simulink model "rocket_6dof_sim"  (R2024a)
settings: Solver=FixedStepAuto  StartTime=0.0  StopTime=35  RelTol=1e-8  AbsTol=1e-8
values from neighbouring files (symbols this model uses):
  p = c(1)+c(2)*tau+c(3)*tau.^2+c(4)*tau.^3+c(5)*tau.^4+c(6)*tau.^5    [envelope_mais_monte_carlo_final.m]    (also in init_mpc.m = falcon9_params(); init_sim.m = falcon9_params(); run_scurve.m = falcon9_params(); simulate_openloop.m = falcon9_params())
  x0_sim = [ic.x0; ic.y0; ic.h0; 0; 0; ic.vz0;                ic.phi0; ic.theta0; 0; 0; ic.q0; 0; ic.m0]    [envelope_mais_monte_carlo_final.m]    (also in init_mpc.m = [p.x0; p.y0; p.h0; init_sim.m = [p.x0)
libraries: simulink_extras x6, simulink x2
settings Model: SimulationMode=accelerator  Creator=marin  LastModifiedBy=marin
settings DataIOCC: SaveFormat=Array
settings OptimizationCC: BlockReduction=off  DefaultParameterBehavior=Inlined  BufferReuse=off

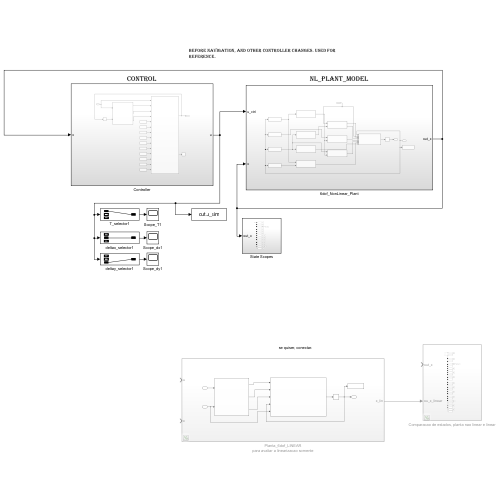
[thumbnail: Simulink's stored preview of the top-level diagram]
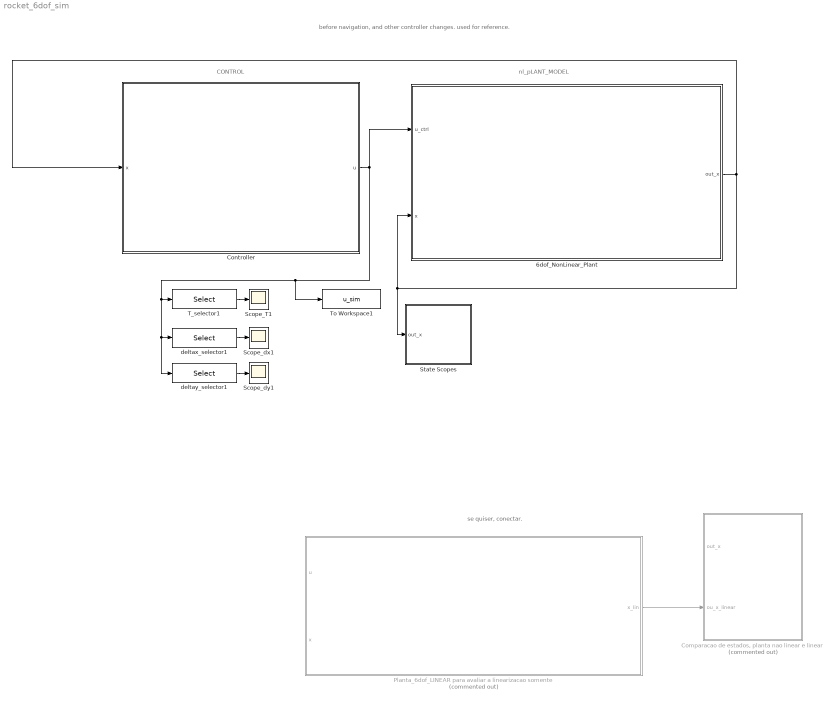
== system rocket_6dof_sim ==
  note: se quiser, conectar.
  note: CONTROL
  note: nl_pLANT_MODEL
  note: before navigation, and other controller changes. used for reference.
  6dof_NonLinear_Plant : Subsystem
  "Comparacao de estados, planta nao linear e linear" : Subsystem  Commented=on
  Controller : Subsystem
  Planta_6dof_LINEAR para avaliar a linearizacao somente : Subsystem  Commented=on
  Scope_T1 : Scope
  Scope_dx1 : Scope
  Scope_dy1 : Scope
  State Scopes : Subsystem
  T_selector1 : Selector  InputPortWidth=3  IndexOptions=Index vector (dialog)  Indices=1  OutputSizes=1
  To Workspace1 : ToWorkspace  VariableName=u_sim  SaveFormat=Timeseries  SampleTime=-1
  deltax_selector1 : Selector  InputPortWidth=3  IndexOptions=Index vector (dialog)  Indices=2  OutputSizes=1
  deltay_selector1 : Selector  InputPortWidth=3  IndexOptions=Index vector (dialog)  Indices=3  OutputSizes=1
  wires:
  deltax_selector1/1 -> Scope_dx1/1
  6dof_NonLinear_Plant/1(out_x) -> Controller/1(x), 6dof_NonLinear_Plant/2(x), State Scopes/1(out_x)
  Controller/1(u) -> 6dof_NonLinear_Plant/1(u_ctrl), deltay_selector1/1, deltax_selector1/1, T_selector1/1, To Workspace1/1
  deltay_selector1/1 -> Scope_dy1/1
  T_selector1/1 -> Scope_T1/1
  Planta_6dof_LINEAR para avaliar a linearizacao somente/1(x_lin) -> "Comparacao de estados, planta nao linear e linear"/2(ou_x_linear)

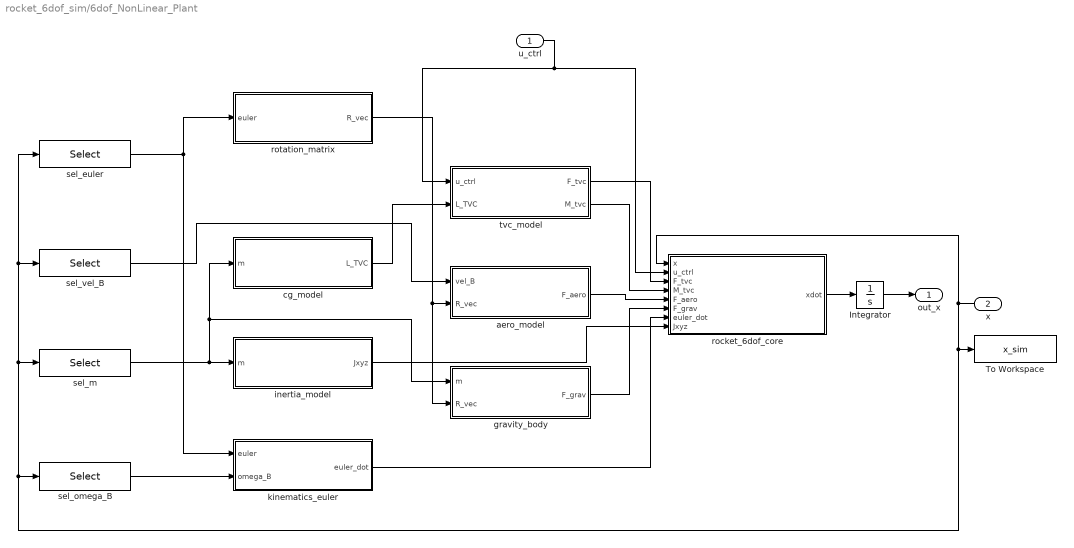
== system rocket_6dof_sim/6dof_NonLinear_Plant ==
  u_ctrl : Inport
  x : Inport  Port=2
  Integrator : Integrator  InitialCondition=x0_sim
  To Workspace : ToWorkspace  VariableName=x_sim  SaveFormat=Timeseries  SampleTime=0.01
  aero_model : MATLAB Function  TreatAsAtomicUnit=on
  cg_model : MATLAB Function  TreatAsAtomicUnit=on
  gravity_body : MATLAB Function  TreatAsAtomicUnit=on
  inertia_model : MATLAB Function  TreatAsAtomicUnit=on
  kinematics_euler : MATLAB Function  TreatAsAtomicUnit=on
  rocket_6dof_core : MATLAB Function  TreatAsAtomicUnit=on
  rotation_matrix : MATLAB Function  TreatAsAtomicUnit=on
  sel_euler : Selector  InputPortWidth=13  IndexOptions=Index vector (dialog)  Indices=7:9  OutputSizes=1
  sel_m : Selector  InputPortWidth=13  IndexOptions=Index vector (dialog)  Indices=13  OutputSizes=1
  sel_omega_B : Selector  InputPortWidth=13  IndexOptions=Index vector (dialog)  Indices=10:12  OutputSizes=1
  sel_vel_B : Selector  InputPortWidth=13  IndexOptions=Index vector (dialog)  Indices=4:6  OutputSizes=1
  tvc_model : MATLAB Function  TreatAsAtomicUnit=on
  out_x : Outport
  wires:
  sel_vel_B/1 -> aero_model/1(vel_B)
  cg_model/1(L_TVC) -> tvc_model/2(L_TVC)
  inertia_model/1(Jxyz) -> rocket_6dof_core/8(Jxyz)
  x/1 -> To Workspace/1, sel_m/1, sel_vel_B/1, sel_euler/1, sel_omega_B/1, rocket_6dof_core/1(x)
  sel_m/1 -> cg_model/1(m), gravity_body/1(m), inertia_model/1(m)
  kinematics_euler/1(euler_dot) -> rocket_6dof_core/7(euler_dot)
  gravity_body/1(F_grav) -> rocket_6dof_core/6(F_grav)
  tvc_model/2(M_tvc) -> rocket_6dof_core/4(M_tvc)
  rotation_matrix/1(R_vec) -> gravity_body/2(R_vec), aero_model/2(R_vec)
  aero_model/1(F_aero) -> rocket_6dof_core/5(F_aero)
  u_ctrl/1 -> rocket_6dof_core/2(u_ctrl), tvc_model/1(u_ctrl)
  tvc_model/1(F_tvc) -> rocket_6dof_core/3(F_tvc)
  Integrator/1 -> out_x/1
  rocket_6dof_core/1(xdot) -> Integrator/1
  sel_omega_B/1 -> kinematics_euler/2(omega_B)
  sel_euler/1 -> rotation_matrix/1(euler), kinematics_euler/1(euler)

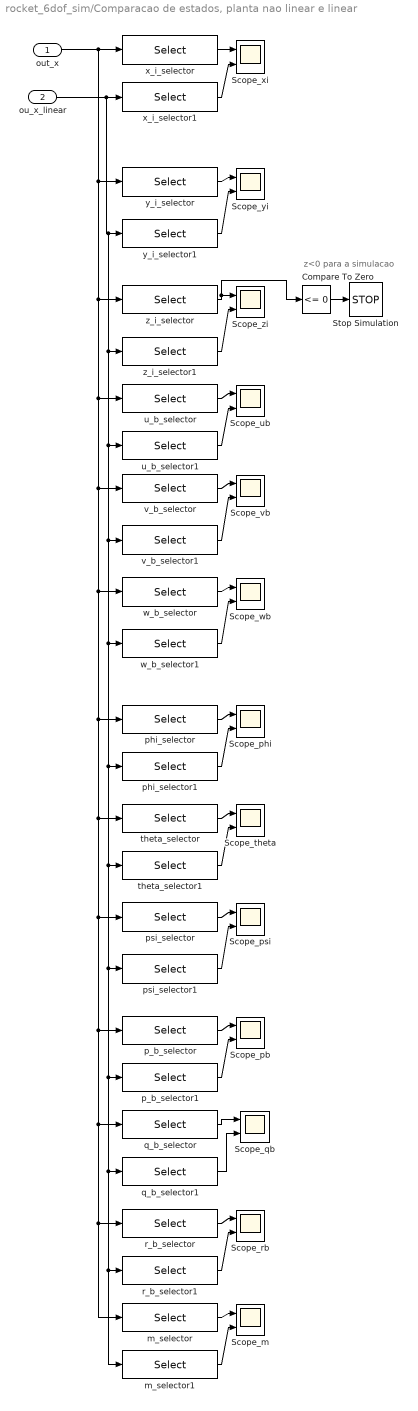
== system rocket_6dof_sim/Comparacao de estados, planta nao linear e linear ==
  note: z<0 para a simulacao
  out_x : Inport
  ou_x_linear : Inport  Port=2
  Compare To Zero : simulink/Logic and Bit Operations/Compare To Zero  relop=<=  OutDataTypeStr=boolean
  Scope_m : Scope  NumInputPorts=2
  Scope_pb : Scope  NumInputPorts=2
  Scope_phi : Scope  NumInputPorts=2
  Scope_psi : Scope  NumInputPorts=2
  Scope_qb : Scope  NumInputPorts=2
  Scope_rb : Scope  NumInputPorts=2
  Scope_theta : Scope  NumInputPorts=2
  Scope_ub : Scope  NumInputPorts=2
  Scope_vb : Scope  NumInputPorts=2
  Scope_wb : Scope  NumInputPorts=2
  Scope_xi : Scope  NumInputPorts=2
  Scope_yi : Scope  NumInputPorts=2
  Scope_zi : Scope  NumInputPorts=2
  Stop Simulation : Stop
  m_selector : Selector  InputPortWidth=13  IndexOptions=Index vector (dialog)  Indices=13  OutputSizes=1
  m_selector1 : Selector  InputPortWidth=13  IndexOptions=Index vector (dialog)  Indices=13  OutputSizes=1
  p_b_selector : Selector  InputPortWidth=13  IndexOptions=Index vector (dialog)  Indices=10  OutputSizes=1
  p_b_selector1 : Selector  InputPortWidth=13  IndexOptions=Index vector (dialog)  Indices=10  OutputSizes=1
  phi_selector : Selector  InputPortWidth=13  IndexOptions=Index vector (dialog)  Indices=7  OutputSizes=1
  phi_selector1 : Selector  InputPortWidth=13  IndexOptions=Index vector (dialog)  Indices=7  OutputSizes=1
  psi_selector : Selector  InputPortWidth=13  IndexOptions=Index vector (dialog)  Indices=9  OutputSizes=1
  psi_selector1 : Selector  InputPortWidth=13  IndexOptions=Index vector (dialog)  Indices=9  OutputSizes=1
  q_b_selector : Selector  InputPortWidth=13  IndexOptions=Index vector (dialog)  Indices=11  OutputSizes=1
  q_b_selector1 : Selector  InputPortWidth=13  IndexOptions=Index vector (dialog)  Indices=11  OutputSizes=1
  r_b_selector : Selector  InputPortWidth=13  IndexOptions=Index vector (dialog)  Indices=12  OutputSizes=1
  r_b_selector1 : Selector  InputPortWidth=13  IndexOptions=Index vector (dialog)  Indices=12  OutputSizes=1
  theta_selector : Selector  InputPortWidth=13  IndexOptions=Index vector (dialog)  Indices=8  OutputSizes=1
  theta_selector1 : Selector  InputPortWidth=13  IndexOptions=Index vector (dialog)  Indices=8  OutputSizes=1
  u_b_selector : Selector  InputPortWidth=13  IndexOptions=Index vector (dialog)  Indices=4  OutputSizes=1
  u_b_selector1 : Selector  InputPortWidth=13  IndexOptions=Index vector (dialog)  Indices=4  OutputSizes=1
  v_b_selector : Selector  InputPortWidth=13  IndexOptions=Index vector (dialog)  Indices=5  OutputSizes=1
  v_b_selector1 : Selector  InputPortWidth=13  IndexOptions=Index vector (dialog)  Indices=5  OutputSizes=1
  w_b_selector : Selector  InputPortWidth=13  IndexOptions=Index vector (dialog)  Indices=6  OutputSizes=1
  w_b_selector1 : Selector  InputPortWidth=13  IndexOptions=Index vector (dialog)  Indices=6  OutputSizes=1
  x_i_selector : Selector  InputPortWidth=13  IndexOptions=Index vector (dialog)  Indices=1  OutputSizes=1
  x_i_selector1 : Selector  InputPortWidth=13  IndexOptions=Index vector (dialog)  Indices=1  OutputSizes=1
  y_i_selector : Selector  InputPortWidth=13  IndexOptions=Index vector (dialog)  Indices=2  OutputSizes=1
  y_i_selector1 : Selector  InputPortWidth=13  IndexOptions=Index vector (dialog)  Indices=2  OutputSizes=1
  z_i_selector : Selector  InputPortWidth=13  IndexOptions=Index vector (dialog)  Indices=3  OutputSizes=1
  z_i_selector1 : Selector  InputPortWidth=13  IndexOptions=Index vector (dialog)  Indices=3  OutputSizes=1
  wires:
  u_b_selector/1 -> Scope_ub/1
  psi_selector/1 -> Scope_psi/1
  y_i_selector/1 -> Scope_yi/1
  q_b_selector/1 -> Scope_qb/1
  p_b_selector/1 -> Scope_pb/1
  phi_selector/1 -> Scope_phi/1
  v_b_selector/1 -> Scope_vb/1
  r_b_selector/1 -> Scope_rb/1
  w_b_selector/1 -> Scope_wb/1
  m_selector/1 -> Scope_m/1
  theta_selector/1 -> Scope_theta/1
  z_i_selector/1 -> Compare To Zero/1, Scope_zi/1
  out_x/1 -> v_b_selector/1, psi_selector/1, p_b_selector/1, q_b_selector/1, r_b_selector/1, m_selector/1, theta_selector/1, phi_selector/1, w_b_selector/1, u_b_selector/1, z_i_selector/1, y_i_selector/1, x_i_selector/1
  Compare To Zero/1 -> Stop Simulation/1
  y_i_selector1/1 -> Scope_yi/2
  z_i_selector1/1 -> Scope_zi/2
  u_b_selector1/1 -> Scope_ub/2
  v_b_selector1/1 -> Scope_vb/2
  w_b_selector1/1 -> Scope_wb/2
  phi_selector1/1 -> Scope_phi/2
  theta_selector1/1 -> Scope_theta/2
  psi_selector1/1 -> Scope_psi/2
  p_b_selector1/1 -> Scope_pb/2
  q_b_selector1/1 -> Scope_qb/2
  r_b_selector1/1 -> Scope_rb/2
  m_selector1/1 -> Scope_m/2
  ou_x_linear/1 -> m_selector1/1, r_b_selector1/1, q_b_selector1/1, p_b_selector1/1, psi_selector1/1, theta_selector1/1, phi_selector1/1, w_b_selector1/1, v_b_selector1/1, u_b_selector1/1, z_i_selector1/1, y_i_selector1/1, x_i_selector1/1
  x_i_selector/1 -> Scope_xi/1
  x_i_selector1/1 -> Scope_xi/2

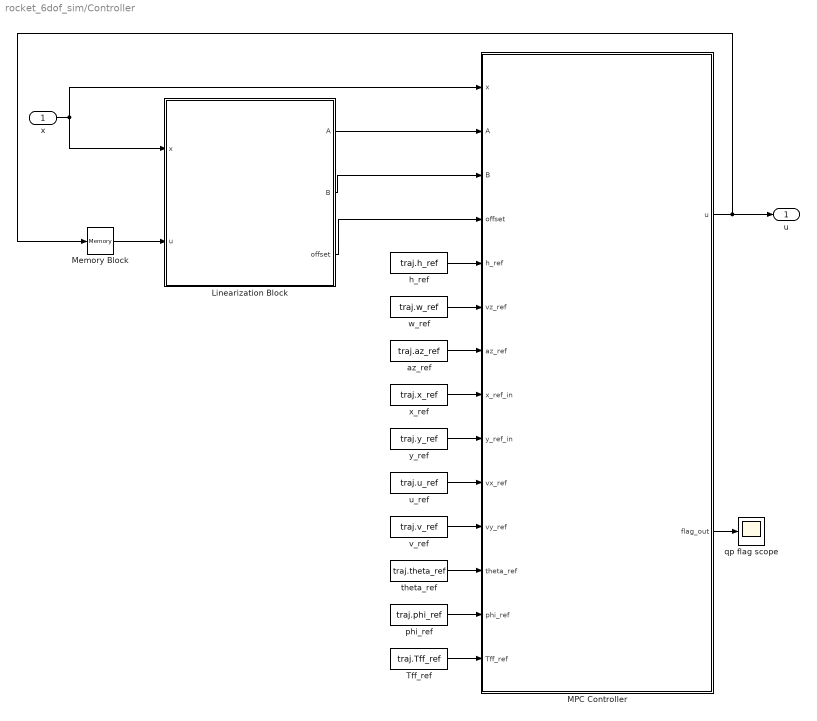
== system rocket_6dof_sim/Controller ==
  x : Inport
  Linearization Block : MATLAB Function  TreatAsAtomicUnit=on  SystemSampleTime=0.01
  MPC Controller : MATLAB Function  TreatAsAtomicUnit=on  SystemSampleTime=0.001
  Memory Block : Memory  InitialCondition=[p.T_min; 0; 0]
  Tff_ref : FromWorkspace  VariableName=traj.Tff_ref  OutputAfterFinalValue=Holding final value
  az_ref : FromWorkspace  VariableName=traj.az_ref  OutputAfterFinalValue=Holding final value
  h_ref : FromWorkspace  VariableName=traj.h_ref  OutputAfterFinalValue=Holding final value
  phi_ref : FromWorkspace  VariableName=traj.phi_ref  OutputAfterFinalValue=Holding final value
  qp flag scope : Scope
  theta_ref : FromWorkspace  VariableName=traj.theta_ref  OutputAfterFinalValue=Holding final value
  u_ref : FromWorkspace  VariableName=traj.u_ref
  v_ref : FromWorkspace  VariableName=traj.v_ref
  w_ref : FromWorkspace  VariableName=traj.w_ref
  x_ref : FromWorkspace  VariableName=traj.x_ref  OutputAfterFinalValue=Holding final value
  y_ref : FromWorkspace  VariableName=traj.y_ref  OutputAfterFinalValue=Holding final value
  u : Outport
  wires:
  y_ref/1 -> MPC Controller/9(y_ref_in)
  theta_ref/1 -> MPC Controller/12(theta_ref)
  Linearization Block/1(A) -> MPC Controller/2(A)
  h_ref/1 -> MPC Controller/5(h_ref)
  phi_ref/1 -> MPC Controller/13(phi_ref)
  MPC Controller/1(u) -> u/1, Memory Block/1
  x_ref/1 -> MPC Controller/8(x_ref_in)
  az_ref/1 -> MPC Controller/7(az_ref)
  Tff_ref/1 -> MPC Controller/14(Tff_ref)
  Linearization Block/2(B) -> MPC Controller/3(B)
  x/1 -> MPC Controller/1(x), Linearization Block/1(x)
  Linearization Block/3(offset) -> MPC Controller/4(offset)
  Memory Block/1 -> Linearization Block/2(u)
  MPC Controller/2(flag_out) -> qp flag scope/1
  u_ref/1 -> MPC Controller/10(vx_ref)
  w_ref/1 -> MPC Controller/6(vz_ref)
  v_ref/1 -> MPC Controller/11(vy_ref)

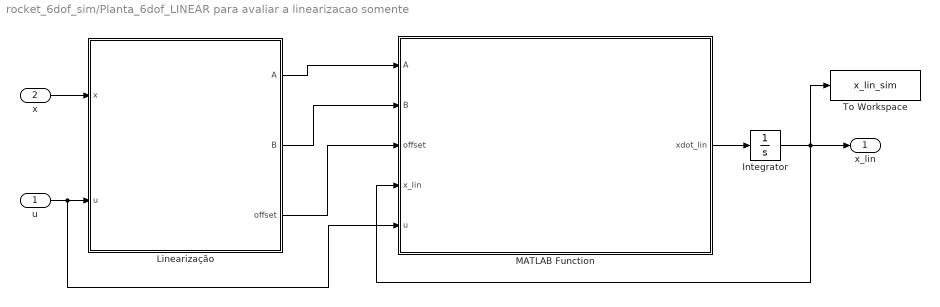
== system rocket_6dof_sim/Planta_6dof_LINEAR para avaliar a linearizacao somente ==
  u : Inport
  x : Inport  Port=2
  Integrator : Integrator  InitialCondition=x0_sim
  Linearização : MATLAB Function  TreatAsAtomicUnit=on  SystemSampleTime=0.3
  MATLAB Function : MATLAB Function  TreatAsAtomicUnit=on
  To Workspace : ToWorkspace  VariableName=x_lin_sim  SaveFormat=Timeseries  SampleTime=0.01
  x_lin : Outport
  wires:
  Linearização/1(A) -> MATLAB Function/1(A)
  Integrator/1 -> To Workspace/1, x_lin/1, MATLAB Function/4(x_lin)
  MATLAB Function/1(xdot_lin) -> Integrator/1
  Linearização/3(offset) -> MATLAB Function/3(offset)
  Linearização/2(B) -> MATLAB Function/2(B)
  u/1 -> MATLAB Function/5(u), Linearização/2(u)
  x/1 -> Linearização/1(x)

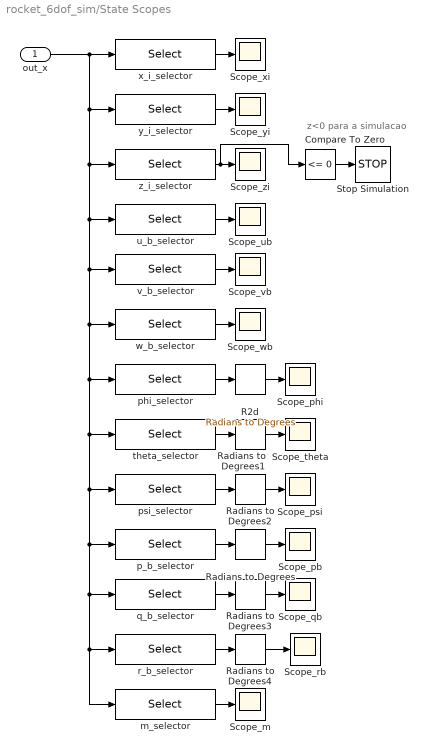
== system rocket_6dof_sim/State Scopes ==
  note: z<0 para a simulacao
  out_x : Inport
  Compare To Zero : simulink/Logic and Bit Operations/Compare To Zero  relop=<=  OutDataTypeStr=boolean
  R2d : simulink_extras/Transformations/Radians to Degrees
  Radians to Degrees{,1..4} (5 alike) : simulink_extras/Transformations/Radians to Degrees
  Scope_m : Scope
  Scope_pb : Scope
  Scope_phi : Scope
  Scope_psi : Scope
  Scope_qb : Scope
  Scope_rb : Scope
  Scope_theta : Scope
  Scope_ub : Scope
  Scope_vb : Scope
  Scope_wb : Scope
  Scope_xi : Scope
  Scope_yi : Scope
  Scope_zi : Scope
  Stop Simulation : Stop
  m_selector : Selector  InputPortWidth=13  IndexOptions=Index vector (dialog)  Indices=13  OutputSizes=1
  p_b_selector : Selector  InputPortWidth=13  IndexOptions=Index vector (dialog)  Indices=10  OutputSizes=1
  phi_selector : Selector  InputPortWidth=13  IndexOptions=Index vector (dialog)  Indices=7  OutputSizes=1
  psi_selector : Selector  InputPortWidth=13  IndexOptions=Index vector (dialog)  Indices=9  OutputSizes=1
  q_b_selector : Selector  InputPortWidth=13  IndexOptions=Index vector (dialog)  Indices=11  OutputSizes=1
  r_b_selector : Selector  InputPortWidth=13  IndexOptions=Index vector (dialog)  Indices=12  OutputSizes=1
  theta_selector : Selector  InputPortWidth=13  IndexOptions=Index vector (dialog)  Indices=8  OutputSizes=1
  u_b_selector : Selector  InputPortWidth=13  IndexOptions=Index vector (dialog)  Indices=4  OutputSizes=1
  v_b_selector : Selector  InputPortWidth=13  IndexOptions=Index vector (dialog)  Indices=5  OutputSizes=1
  w_b_selector : Selector  InputPortWidth=13  IndexOptions=Index vector (dialog)  Indices=6  OutputSizes=1
  x_i_selector : Selector  InputPortWidth=13  IndexOptions=Index vector (dialog)  Indices=1  OutputSizes=1
  y_i_selector : Selector  InputPortWidth=13  IndexOptions=Index vector (dialog)  Indices=2  OutputSizes=1
  z_i_selector : Selector  InputPortWidth=13  IndexOptions=Index vector (dialog)  Indices=3  OutputSizes=1
  wires:
  u_b_selector/1 -> Scope_ub/1
  y_i_selector/1 -> Scope_yi/1
  v_b_selector/1 -> Scope_vb/1
  x_i_selector/1 -> Scope_xi/1
  w_b_selector/1 -> Scope_wb/1
  m_selector/1 -> Scope_m/1
  z_i_selector/1 -> Compare To Zero/1, Scope_zi/1
  out_x/1 -> v_b_selector/1, m_selector/1, r_b_selector/1, q_b_selector/1, p_b_selector/1, psi_selector/1, theta_selector/1, phi_selector/1, w_b_selector/1, u_b_selector/1, z_i_selector/1, y_i_selector/1, x_i_selector/1
  Compare To Zero/1 -> Stop Simulation/1
  phi_selector/1 -> R2d/1
  R2d/1 -> Scope_phi/1
  theta_selector/1 -> Radians to Degrees1/1
  Radians to Degrees1/1 -> Scope_theta/1
  psi_selector/1 -> Radians to Degrees2/1
  Radians to Degrees2/1 -> Scope_psi/1
  p_b_selector/1 -> Radians to Degrees/1
  Radians to Degrees/1 -> Scope_pb/1
  q_b_selector/1 -> Radians to Degrees3/1
  Radians to Degrees3/1 -> Scope_qb/1
  Radians to Degrees4/1 -> Scope_rb/1
  r_b_selector/1 -> Radians to Degrees4/1

== matlab function rocket_6dof_sim/Planta_6dof_LINEAR para avaliar a linearizacao somente/Linearização ==
  data: x input; u input; A output; B output; offset output
function [A, B, offset] = linearizar_planta(x, u)
% LINEARIZAR_PLANTA  Linearização numérica em tempo real da planta 6-DOF.
%
% Bloco MATLAB Function no Simulink.
% Cola este código diretamente dentro do bloco (duplo-clique → editor).
%
% ── O QUE FAZ ────────────────────────────────────────────────────────────
%
%   Dado o estado atual x [13×1] e a entrada atual u [3×1], calcula:
%
%     A      [13×13] — Jacobiana ∂f/∂x
%     B      [13×3]  — Jacobiana ∂f/∂u
%     offset [13×1]  — termo afim da linearização
%
%   Modelo linear resultante (forma afim do espaço de estados):
%
%       ẋ_lin = A · x_lin + B · u + offset
%
%   onde:
%       offset = f(x₀, u₀) − A·x₀ − B·u₀
%
%   Os 13 estados são:
%     x(1:3)   — posição inercial [m]
%     x(4:6)   — velocidade no corpo [m/s]
%     x(7:9)   — ângulos de Euler [rad]
%     x(10:12) — taxas angulares [rad/s]
%     x(13)    — massa [kg]
%
% ── ENTRADAS (portas do bloco Simulink) ──────────────────────────────────
%
%   x  [13×1] — estado atual da planta NÃO-LINEAR
%   u  [3×1]  — entrada de controle atual [T; delta_y; delta_z]
%
% ── SAÍDAS (portas do bloco Simulink) ────────────────────────────────────
%
%   A      [13×13] — Jacobiana dos estados
%   B      [13×3]  — Jacobiana das entradas
%   offset [13×1]  — termo afim (gravidade, bias, etc.)
%
% Matheus Martins Marinato — TCC UFSM 2025/2026

%#codegen
coder.extrinsic('rocket_6dof', 'falcon9_params');

persistent p
if isempty(p)
    p = falcon9_params();
end

% ── Dimensões ──
nx = 13;   % todos os estados, incluindo massa
nu = 3;

% ── Pré-alocação ──
A      = zeros(nx, nx);
B      = zeros(nx, nu);
offset = zeros(nx, 1);

% ── Perturbações por tipo de variável ──
dx = [1e-2;  ... %  1. x_I   [m]
      1e-2;  ... %  2. y_I   [m]
      1e-2;  ... %  3. z_I   [m]
      1e-2;  ... %  4. u_B   [m/s]
      1e-2;  ... %  5. v_B   [m/s]
      1e-2;  ... %  6. w_B   [m/s]
      1e-4;  ... %  7. phi   [rad]
      1e-4;  ... %  8. theta [rad]
      1e-4;  ... %  9. psi   [rad]
      1e-4;  ... % 10. p_B   [rad/s]
      1e-4;  ... % 11. q_B   [rad/s]
      1e-4;  ... % 12. r_B   [rad/s]
      1.0];      % 13. m     [kg]

du = [100;   ... % T       [N]
      1e-5;  ... % delta_y [rad]
      1e-5];     % delta_z [rad]

t = 0;

% ── f₀: derivada no ponto de operação ──
f0 = zeros(nx, 1);
f0 = rocket_6dof(t, x, u, p);

% ── Jacobiana A = ∂f/∂x ──
for i = 1:nx
    x_plus      = x;
    x_minus     = x;
    x_plus(i)   = x(i) + dx(i);
    x_minus(i)  = x(i) - dx(i);

    f_plus  = zeros(nx, 1);
    f_minus = zeros(nx, 1);
    f_plus  = rocket_6dof(t, x_plus,  u, p);
    f_minus = rocket_6dof(t, x_minus, u, p);

    A(:, i) = (f_plus - f_minus) / (2 * dx(i));
end

% ── Jacobiana B = ∂f/∂u ──
for j = 1:nu
    u_plus      = u;
    u_minus     = u;
    u_plus(j)   = u(j) + du(j);
    u_minus(j)  = u(j) - du(j);

    f_plus  = zeros(nx, 1);
    f_minus = zeros(nx, 1);
    f_plus  = rocket_6dof(t, x, u_plus,  p);
    f_minus = rocket_6dof(t, x, u_minus, p);

    B(:, j) = (f_plus - f_minus) / (2 * du(j));
end

% ── Offset (termo afim C) ───────────────────────────────────────────────
%
%   ẋ = A·x + B·u + C    onde   C = f₀ − A·x₀ − B·u₀

offset = f0 - A * x - B * u;

end

== matlab function rocket_6dof_sim/Planta_6dof_LINEAR para avaliar a linearizacao somente/MATLAB Function ==
  data: A input; B input; offset input; x_lin input; u input; xdot_lin output
function xdot_lin = planta_linearizada(A, B, offset, x_lin, u)
% PLANTA_LINEARIZADA  Modelo linear 13 estados, independente.
%
% Bloco MATLAB Function no Simulink.
% Cola este código diretamente dentro do bloco (duplo-clique → editor).
%
% ── EQUAÇÃO ──────────────────────────────────────────────────────────────
%
%       ẋ_lin = A · x_lin + B · u + offset
%
%   13 estados completos (posição, velocidade, atitude, taxas, massa).
%   Não depende de x_nl. Roda com seu próprio integrador e CI.
%
% ── ENTRADAS ─────────────────────────────────────────────────────────────
%
%   A      [13×13] — do bloco linearizar_planta
%   B      [13×3]  — do bloco linearizar_planta
%   offset [13×1]  — do bloco linearizar_planta
%   x_lin  [13×1]  — feedback do seu próprio integrador
%   u      [3×1]   — entrada de controle
%
% ── SAÍDA ────────────────────────────────────────────────────────────────
%
%   xdot_lin [13×1] — derivada → vai pro integrador da planta linear
%
% Matheus Martins Marinato — TCC UFSM 2025/2026

%#codegen

xdot_lin = A * x_lin + B * u + offset;

end

== matlab function rocket_6dof_sim/6dof_NonLinear_Plant/aero_model ==
  data: vel_B input; F_aero output; R_vec input
function F_aero = fcn(vel_B, R_vec)
% hardcoded aqui no bloco (identico ao .m correspondente),
% para evitar coder.extrinsic, que estava reclamando 
rho = 1.225;  Sref = 10.52;  CD0 = 0.30;

R_IB  = reshape(R_vec, 3, 3);
v_rel = vel_B;   % vento = 0 nominal
v_mag = norm(v_rel);
if v_mag < 1e-6
    F_aero = zeros(3,1);
else
    D      = 0.5 * rho * v_mag^2 * Sref * CD0;
    F_aero = -D * (v_rel / v_mag);
end

== matlab function rocket_6dof_sim/6dof_NonLinear_Plant/cg_model ==
  data: m input; L_TVC output
function L_TVC = fcn(m)
% hardcoded aqui no bloco (identico ao .m correspondente),
% para evitar coder.extrinsic, que estava reclamando 
r_CG_0 = 18.5;   r_CG_f = 17.0;
m0 = 30000;       mf = 22500;

frac  = max(0, min(1, (m - mf) / (m0 - mf)));
L_TVC = r_CG_f + (r_CG_0 - r_CG_f) * frac;

== matlab function rocket_6dof_sim/6dof_NonLinear_Plant/gravity_body ==
  data: m input; F_grav output; R_vec input
function F_grav = fcn(m, R_vec)
g    = 9.80665;
R_IB = reshape(R_vec, 3, 3);
F_grav = m * (R_IB' * [0; 0; -g]);

== matlab function rocket_6dof_sim/6dof_NonLinear_Plant/inertia_model ==
  data: m input; Jxyz output
function Jxyz = fcn(m)
% hardcoded aqui no bloco (identico ao .m correspondente),
% para evitar coder.extrinsic, que estava reclamando 
m0 = 30000;  mf = 22500;
Jzz0 = 8.741e4;  Jzz_f = 7.485e4;
Jxx0 = 3.805e6;  Jxx_f = 3.202e6;

frac = max(0, min(1, (m - mf) / (m0 - mf)));
Jzz  = Jzz_f + (Jzz0 - Jzz_f) * frac;
Jxx  = Jxx_f + (Jxx0 - Jxx_f) * frac;
Jxyz = [Jxx; Jxx; Jzz];  % [Jxx; Jyy=Jxx; Jzz]

== matlab function rocket_6dof_sim/6dof_NonLinear_Plant/kinematics_euler ==
  data: euler input; euler_dot output; omega_B input
function euler_dot = fcn(euler, omega_B)
% Chama kinematics_euler.m
euler_dot = kinematics_euler(euler, omega_B);

== matlab function rocket_6dof_sim/6dof_NonLinear_Plant/rocket_6dof_core ==
  data: x input; xdot output; u_ctrl input; F_tvc input; M_tvc input; F_aero input; F_grav input; euler_dot input; Jxyz input
function xdot = fcn(x, u_ctrl, F_tvc, M_tvc, F_aero, F_grav, euler_dot, Jxyz)
% Montagem final das EDOs 6-DOF. Forças, momentos, euler_dot e inércia
% chegam prontos de blocos a montante; aqui só monta Newton-Euler.
% hardcoded aqui no bloco (identico ao .m correspondente),
% para evitar coder.extrinsic, que estava reclamando
T_max = 845000;  T_min = 338000;
Isp = 282;       g0 = 9.80665;   mf = 22500;
vel_B   = x(4:6);
euler   = x(7:9);
omega_B = x(10:12);
m       = max(mf, x(13));
T       = max(T_min, min(T_max, u_ctrl(1)));
% R_IB
phi=euler(1); theta=euler(2); psi=euler(3);
R_IB = rotation_matrix(phi, theta, psi);
% EQ
pos_dot = R_IB * vel_B;
% EQ
F_total = F_tvc + F_aero + F_grav;
vel_dot = (1/m)*F_total - cross(omega_B, vel_B);   % Coriolis no corpo
% EQ
Jxx=Jxyz(1); Jyy=Jxyz(2); Jzz=Jxyz(3);
J    = diag([Jxx; Jyy; Jzz]);
Jinv = diag([1/Jxx; 1/Jyy; 1/Jzz]);
omega_dot = Jinv*(M_tvc - cross(omega_B, J*omega_B));   % termo giroscopico
% EQ
if x(13) > mf + 1.0    % margem evita oscilar massa em torno de mf
    m_dot = -T/(Isp*g0);
else
    m_dot = 0;
end
xdot = [pos_dot; vel_dot; euler_dot; omega_dot; m_dot];

== matlab function rocket_6dof_sim/6dof_NonLinear_Plant/rotation_matrix ==
  data: euler input; R_vec output
function R_vec = fcn(euler)
% Chama rotation_matrix.m -> achata 3x3 para 9x1
R     = rotation_matrix(euler(1), euler(2), euler(3));
R_vec = R(:);

== matlab function rocket_6dof_sim/6dof_NonLinear_Plant/tvc_model ==
  data: u_ctrl input; F_tvc output; L_TVC input; M_tvc output
function [F_tvc, M_tvc] = fcn(u_ctrl, L_TVC)
% Chama tvc_model.m  |  u_ctrl = [T; delta_y; delta_x]
[F_tvc, M_tvc] = tvc_model(u_ctrl(1), u_ctrl(2), u_ctrl(3), L_TVC);

== matlab function rocket_6dof_sim/Controller/Linearization Block ==
  data: x input; u input; A output; B output; offset output
function [A, B, offset] = linearizar_planta(x, u)
%#codegen
% Lineariza rocket_6dof em torno de (x,u) por diferenças finitas centradas.
% Modelo afim resultante: x_dot = A*x + B*u + offset, com A=df/dx, B=df/du.
% Recalculado a cada passo do LTV-MPC (o ponto de operação muda durante a descida).
coder.extrinsic('rocket_6dof', 'falcon9_params', 'evalin');

% p e T_min só precisam ser lidos uma vez; persistent evita refazer a cada chamada.
persistent p T_min_lin
if isempty(p)
    p = falcon9_params();
    T_min_lin = 0;
    T_min_lin = evalin('base', 'p.T_min');
end
nx = 13;
nu = 3;
A      = zeros(nx, nx);
B      = zeros(nx, nu);
offset = zeros(nx, 1);
% ── Garantir u dentro do envelope do motor ──────────────────────────────
%   Durante queda livre, u(1)=0 chega via Memory.
%   A linearização precisa de T >= T_min pra que as perturbações +-delta
%   não sejam ambas saturadas pro mesmo valor (o que zeraria a coluna de B).
u_lin = u;
if u_lin(1) < T_min_lin
    u_lin(1) = T_min_lin;
end
% Passo de cada perturbação. Estados de posição/velocidade toleram passo
% maior; ângulos/taxas usam 1e-4 (sensíveis); massa usa 1 kg (escala grande).
% du do empuxo é 100 N (T é da ordem de 1e5); TVC usa 1e-5 rad.
dx = [1e-2; 1e-2; 1e-2;
      1e-2; 1e-2; 1e-2;
      1e-4; 1e-4; 1e-4;
      1e-4; 1e-4; 1e-4;
      1.0];
du = [100; 1e-5; 1e-5];
t = 0;
% f0: derivada no ponto de operação. zeros(...) antes da chamada é exigência
% do codegen, rocket_6dof é extrínseca, então o tipo da saída tem que ser
% pré-declarado (mesmo padrão em todas as chamadas abaixo).
f0 = zeros(nx, 1);
f0 = rocket_6dof(t, x, u_lin, p);
% A = df/dx coluna a coluna: perturba só o estado i, mantém u fixo.
for i = 1:nx
    x_plus      = x;
    x_minus     = x;
    x_plus(i)   = x(i) + dx(i);
    x_minus(i)  = x(i) - dx(i);
    f_plus  = zeros(nx, 1);
    f_minus = zeros(nx, 1);
    f_plus  = rocket_6dof(t, x_plus,  u_lin, p);
    f_minus = rocket_6dof(t, x_minus, u_lin, p);
    A(:, i) = (f_plus - f_minus) / (2 * dx(i));
end
% B = df/du: mesma coisa, perturbando entrada j com x fixo.
for j = 1:nu
    u_plus      = u_lin;
    u_minus     = u_lin;
    u_plus(j)   = u_lin(j) + du(j);
    u_minus(j)  = u_lin(j) - du(j);
    f_plus  = zeros(nx, 1);
    f_minus = zeros(nx, 1);
    f_plus  = rocket_6dof(t, x, u_plus,  p);
    f_minus = rocket_6dof(t, x, u_minus, p);
    B(:, j) = (f_plus - f_minus) / (2 * du(j));
end
% Termo afim que faz o modelo bater com f0 no ponto de operação.
offset = f0 - A * x - B * u_lin;
end

== matlab function rocket_6dof_sim/Controller/MPC Controller ==
  data: x input; u output; A input; B input; offset input; h_ref input; vz_ref input; az_ref input; x_ref_in input; y_ref_in input; vx_ref input; vy_ref input; theta_ref input; phi_ref input; Tff_ref input; flag_out output
function [u, flag_out] = controlador_mpc(x, A, B, offset, h_ref, vz_ref, az_ref, ...
                              x_ref_in, y_ref_in, vx_ref, vy_ref, ...
                              theta_ref, phi_ref, Tff_ref)
% CONTROLADOR_MPC  LTV-MPC com feedforward, ímã de proximidade e tracking
%
%   Error-State MPC: otimiza correções ΔU em torno do empuxo feedforward.
%   Referências vindas da S-Curve 3D (Guidance).
%
%   Entradas:
%     x          - Estado atual da planta [13×1]
%     A, B       - Matrizes linearizadas (atualizadas a cada 0.3s)
%     offset     - Termo afim da linearização (não usado aqui, mas disponível)
%     h_ref, vz_ref, az_ref  - Referências verticais da S-curve
%     x_ref_in, y_ref_in     - Referências de posição lateral
%     vx_ref, vy_ref         - Referências de velocidade lateral
%     theta_ref, phi_ref     - Referências de atitude (inclinação comandada)
%     Tff_ref                - Empuxo feedforward da S-curve [N]
%
%   Saídas:
%     u          - Comando [T; δy; δx]
%     flag_out   - exitflag do quadprog (>0 = convergiu)

%#codegen
coder.extrinsic('quadprog', 'evalin');

% ── Pré-alocação das saídas ─────────────────────────────────────────────
u = zeros(3,1);
flag_out = 1;

% ── Variáveis persistentes (carregadas uma vez) ─────────────────────────
persistent T_min T_max delta_max m0_ref ...
           Ts Np Nc nx nu N_skip ...
           Q_w R_w ...
           u_held step_cnt idx inicializado

if isempty(inicializado)
    T_min     = 0;  T_min     = evalin('base', 'p.T_min');
    T_max     = 0;  T_max     = evalin('base', 'p.T_max');
    delta_max = 0;  delta_max = evalin('base', 'p.delta_max');
    m0_ref    = 0;  m0_ref    = evalin('base', 'p.m0');

    % Parâmetros do MPC
    Ts     = 0.1;     % [s] Período de amostragem do MPC
    Np     = 35;      % [-] Horizonte de predição (3.5s)
    Nc     = 3;       % [-] Horizonte de controle (3 moves livres)
    nx     = 10;      % [-] Estados de erro (pos3, vel3, phi, theta, p, q)
    nu     = 3;       % [-] Entradas (T, δy, δx)
    N_skip = 100;     % [-] Simulink steps entre resoluções do QP (0.1s a 1kHz)

    % Pesos Q e R (Bryson × multiplicadores, definidos no init_mpc.m)
    Q_w = zeros(10,10); Q_w = evalin('base', 'Q_mpc');
    R_w = zeros(3,3);   R_w = evalin('base', 'R_mpc');

    % Índices dos 10 estados usados (exclui psi, r_B e m do vetor x[13])
    idx = [1,2,3, 4,5,6, 7,8, 10,11];

    u_held   = zeros(3,1);
    step_cnt = 0;
    inicializado = true;
end

% ═════════════════════════════════════════════════════════════════════════
%  BYPASS DE QUEDA LIVRE
%  Enquanto a S-curve não comanda motor, saída zero.
% ═════════════════════════════════════════════════════════════════════════
if Tff_ref <= (T_min + 1.0)
    u_held = u;
    step_cnt = 0;
    return;
end

% ═════════════════════════════════════════════════════════════════════════
%  SAMPLE-AND-HOLD
%  Resolve QP a cada N_skip steps; mantém comando constante entre eles.
% ═════════════════════════════════════════════════════════════════════════
step_cnt = mod(step_cnt, N_skip) + 1;
if step_cnt ~= 1
    u = u_held;
    return;
end

% ═════════════════════════════════════════════════════════════════════════
%  VETOR DE ERRO (Error-State)
%  e = x_atual - x_referência
% ═════════════════════════════════════════════════════════════════════════
x10 = x(idx);

x_ref = zeros(nx, 1);
x_ref(1)  = x_ref_in;     % x_I  [m]
x_ref(2)  = y_ref_in;     % y_I  [m]
x_ref(3)  = h_ref;        % z_I  [m]
x_ref(4)  = vx_ref;       % u_B  [m/s]
x_ref(5)  = vy_ref;       % v_B  [m/s]
x_ref(6)  = vz_ref;       % w_B  [m/s]
x_ref(7)  = phi_ref;      % φ    [rad]  (inclinação comandada pelo Guidance)
x_ref(8)  = theta_ref;    % θ    [rad]
x_ref(9)  = 0;            % p_B  [rad/s]
x_ref(10) = 0;            % q_B  [rad/s]

e0 = x10 - x_ref;

% ═════════════════════════════════════════════════════════════════════════
%  FEEDFORWARD
%  Empuxo base vindo da S-curve, escalado pela massa real.
%  O QP otimiza ΔU em torno deste ponto.
% ═════════════════════════════════════════════════════════════════════════
u_ff = zeros(nu, 1);
u_ff(1) = Tff_ref * (x(13) / m0_ref);
u_ff(1) = max(T_min, min(T_max, u_ff(1)));

% ═════════════════════════════════════════════════════════════════════════
%  DISCRETIZAÇÃO E MATRIZES DE PREDIÇÃO
%  Euler explícito: Ad = I + A·Ts,  Bd = B·Ts
%  Phi  (Np·nx × nx)    : propaga o erro livre (sem controle)
%  Gamma(Np·nx × Nc·nu) : mapeia cada move ΔU no erro futuro
% ═════════════════════════════════════════════════════════════════════════
A10 = A(idx, idx);
B10 = B(idx, 1:3);
Ad  = eye(nx) + A10 * Ts;
Bd  = B10 * Ts;

Phi   = zeros(Np*nx, nx);
Gamma = zeros(Np*nx, Nc*nu);
Ad_pow = eye(nx);

for i = 1:Np
    Ad_pow = Ad_pow * Ad;
    ri = (i-1)*nx + 1 : i*nx;
    Phi(ri, :) = Ad_pow;
end

for j = 1:Nc
    cj = (j-1)*nu + 1 : j*nu;
    if j < Nc
        % Moves 1 e 2: comando aplicado uma vez no step j e mantido
        Ad_p = eye(nx);
        for i = j:Np
            ri = (i-1)*nx + 1 : i*nx;
            Gamma(ri, cj) = Ad_p * Bd;
            Ad_p = Ad_p * Ad;
        end
    else
        % Move 3 (último): mantido constante até o fim do horizonte
        % Acumula efeito composto (soma de contribuições)
        Ad_p = eye(nx);
        acc  = zeros(nx, nu);
        for i = j:Np
            acc = acc + Ad_p * Bd;
            ri  = (i-1)*nx + 1 : i*nx;
            Gamma(ri, cj) = acc;
            Ad_p = Ad_p * Ad;
        end
    end
end

% ═════════════════════════════════════════════════════════════════════════
%  MONTAGEM DO CUSTO
%  Q_bar: penalidade nos erros ao longo do horizonte
%  Q_terminal: penalidade reforçada no último step (Ímã de Proximidade)
% ═════════════════════════════════════════════════════════════════════════
Q_bar = zeros(Np*nx, Np*nx);
for i = 1:(Np-1)
    ri = (i-1)*nx + 1 : i*nx;
    Q_bar(ri, ri) = Q_w;
end

% ── Ímã de Proximidade Dinâmica ──────────────────────────────────────────
% Abaixo de 80m, escala os pesos terminais de posição (x,y,z) e
% velocidade vertical (w_B) de 1× até 100×. Prioriza a "foto final"
% nos metros decisivos, onde perturbações residuais não têm tempo de
% ser corrigidas de outra forma.
h_atual      = x10(3);
h_inicio_ima = 80.0;

if h_atual > h_inicio_ima
    Fator_Urgencia = 1.0;
else
    alpha_ima = (h_inicio_ima - h_atual) / h_inicio_ima;
    Fator_Urgencia = 1.0 + 99.0 * alpha_ima;
end

Q_terminal = Q_w;
Q_terminal(1,1) = Q_w(1,1) * Fator_Urgencia;  % x_I
Q_terminal(2,2) = Q_w(2,2) * Fator_Urgencia;  % y_I
Q_terminal(3,3) = Q_w(3,3) * Fator_Urgencia;  % z_I
Q_terminal(6,6) = Q_w(6,6) * Fator_Urgencia;  % w_B

ri_last = (Np-1)*nx + 1 : Np*nx;
Q_bar(ri_last, ri_last) = Q_terminal;

% ── Custo no esforço de controle (R_bar) ─────────────────────────────────
R_bar = zeros(Nc*nu, Nc*nu);
for j = 1:Nc
    cj = (j-1)*nu + 1 : j*nu;
    R_bar(cj, cj) = R_w;
end

% ═════════════════════════════════════════════════════════════════════════
%  FORMULAÇÃO QP
%  J = ΔU'·H·ΔU + f'·ΔU   →   min com quadprog
% ═════════════════════════════════════════════════════════════════════════
GtQ  = Gamma' * Q_bar;
H_qp = 2.0 * (GtQ * Gamma + R_bar);
f_qp = 2.0 * (GtQ * Phi * e0);
H_qp = 0.5 * (H_qp + H_qp');          % Garante simetria numérica

% ── Restrições de box (relativas ao feedforward) ────────────────────────
lb_dU = zeros(Nc*nu, 1);
ub_dU = zeros(Nc*nu, 1);
for j = 1:Nc
    base = (j-1)*nu;
    lb_dU(base+1) = T_min     - u_ff(1);    % Quanto posso reduzir T
    lb_dU(base+2) = -delta_max - u_ff(2);
    lb_dU(base+3) = -delta_max - u_ff(3);

    ub_dU(base+1) = T_max     - u_ff(1);    % Quanto posso aumentar T
    ub_dU(base+2) =  delta_max - u_ff(2);
    ub_dU(base+3) =  delta_max - u_ff(3);
end

% ═════════════════════════════════════════════════════════════════════════
%  RESOLVER QP
% ═════════════════════════════════════════════════════════════════════════
dU_opt   = zeros(Nc*nu, 1);
fval     = 0;
exitflag = 0;

[dU_opt, fval, exitflag] = quadprog(H_qp, f_qp, [], [], [], [], ...
                                    lb_dU, ub_dU, zeros(Nc*nu,1), ...
                                    evalin('base', 'opts_qp'));

% ═════════════════════════════════════════════════════════════════════════
%  COMANDO FINAL
%  Se QP convergiu: u = feedforward + correção
%  Se falhou:       u = feedforward puro (fallback seguro)
% ═════════════════════════════════════════════════════════════════════════
if exitflag > 0
    u(1) = u_ff(1) + dU_opt(1);
    u(2) = u_ff(2) + dU_opt(2);
    u(3) = u_ff(3) + dU_opt(3);
else
    u(1) = u_ff(1);
    u(2) = u_ff(2);
    u(3) = u_ff(3);
end

% Saturação de segurança (redundante, QP já respeita, mas protege contra
% erros numéricos ou fallback)
u(1) = max(T_min,      min(T_max,      u(1)));
u(2) = max(-delta_max,  min(delta_max,  u(2)));
u(3) = max(-delta_max,  min(delta_max,  u(3)));

u_held   = u;
flag_out = exitflag;
end
